simulink model "accelerometer02"  (R2016b)
settings: Solver=FixedStepAuto  StartTime=0.0  StopTime=inf  RelTol=1e-3
libraries: simulink_extras x2, androidlib x1
settings Model: SimulationMode=external  Creator=vibek  LastModifiedBy=vibek
settings OptimizationCC: MaxStackSize=64
settings DebuggingCC: ParameterTunabilityLossMsg=error
settings HardwareCC: ProdBitPerPointer=32  ProdBitPerSizeT=32  ProdBitPerPtrDiffT=32  ProdLargestAtomicInteger=Long  ProdLargestAtomicFloat=Double  ProdWordSize=32  ProdHWDeviceType=ARM Compatible->ARM Cortex  UseEmbeddedCoderFeatures=off  UseSimulinkCoderFeatures=off
settings RTWCC: SystemTargetFile=ert.tlc  HardwareBoard=Android Device  TLCOptions="-aInlineSetEventsForThisBaseRateFcn=TLC_FALSE -aSuppressMultiTaskScheduler=TLC_FALSE  -aRateBasedStepFcn=0"  TemplateMakefile=ert_default_tmf  Description=Embedded Coder  GenerateReport=on  Toolchain=Android SDK/NDK Tools  LaunchReport=on
settings CodeAppCC: ForceParamTrailComments=on  OperatorAnnotations=on  MATLABSourceComments=on
settings ERTTargetCC: ERTCustomFileBanners=off  SupportContinuousTime=on  SupportNonInlinedSFcns=on  RemoveResetFunc=off  ModelStepFunctionPrototypeControlCompliant=off

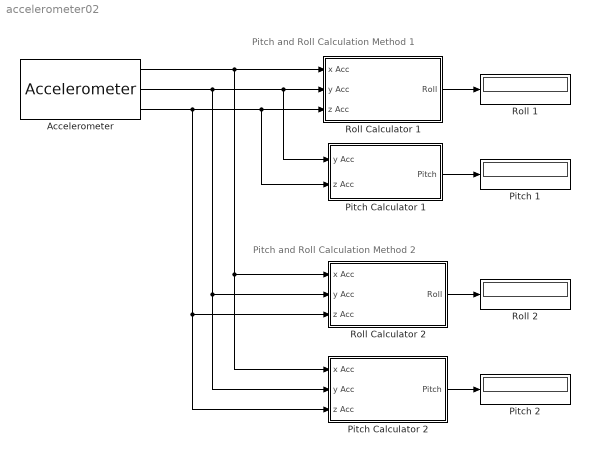
== system accelerometer02 ==
  note: Pitch and Roll Calculation Method 2
  note: Pitch and Roll Calculation Method 1
  Accelerometer : androidlib/Accelerometer  OutputVector=off  SampleTime=0.1  BlockPlatform=Android
  Pitch 1 : Display
      settings: Decimation=5
  Pitch 2 : Display
      settings: Decimation=6
  Pitch Calculator 1 : Subsystem
  Pitch Calculator 2 : Subsystem
  Roll 1 : Display
      settings: Decimation=5
  Roll 2 : Display
      settings: Decimation=6
  Roll Calculator 1 : Subsystem
  Roll Calculator 2 : Subsystem
  wires:
  Roll Calculator 1/1(Roll) -> Roll 1/1
  Pitch Calculator 1/1(Pitch) -> Pitch 1/1
  Accelerometer/1 -> Pitch Calculator 2/1(x Acc), Roll Calculator 2/1(x Acc), Roll Calculator 1/1(x Acc)
  Accelerometer/2 -> Pitch Calculator 2/2(y Acc), Roll Calculator 2/2(y Acc), Pitch Calculator 1/1(y Acc), Roll Calculator 1/2(y Acc)
  Accelerometer/3 -> Pitch Calculator 2/3(z Acc), Roll Calculator 2/3(z Acc), Pitch Calculator 1/2(z Acc), Roll Calculator 1/3(z Acc)
  Pitch Calculator 2/1(Pitch) -> Pitch 2/1
  Roll Calculator 2/1(Roll) -> Roll 2/1

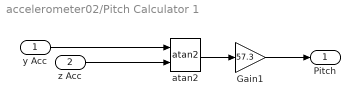
== system accelerometer02/Pitch Calculator 1 ==
  y Acc : Inport
  z Acc : Inport  Port=2
  Gain1 : Gain  Gain=57.3
  atan2 : Trigonometry  Operator=atan2
  Pitch : Outport
  wires:
  Gain1/1 -> Pitch/1
  atan2/1 -> Gain1/1
  y Acc/1 -> atan2/1
  z Acc/1 -> atan2/2

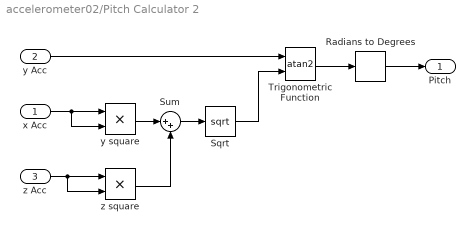
== system accelerometer02/Pitch Calculator 2 ==
  x Acc : Inport
  y Acc : Inport  Port=2
  z Acc : Inport  Port=3
  Radians to Degrees : simulink_extras/Transformations/Radians to Degrees
  Sqrt : Sqrt  SaturateOnIntegerOverflow=on
  Sum : Sum  Inputs=|++
  Trigonometric Function : Trigonometry  Operator=atan2
  y square : Product
  z square : Product
  Pitch : Outport
  wires:
  Radians to Degrees/1 -> Pitch/1
  Trigonometric Function/1 -> Radians to Degrees/1
  Sqrt/1 -> Trigonometric Function/2
  z square/1 -> Sum/2
  Sum/1 -> Sqrt/1
  z Acc/1 -> z square/1, z square/2
  y Acc/1 -> Trigonometric Function/1
  x Acc/1 -> y square/2, y square/1
  y square/1 -> Sum/1

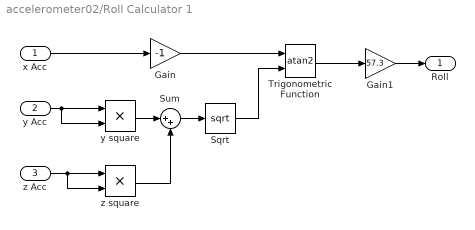
== system accelerometer02/Roll Calculator 1 ==
  x Acc : Inport
  y Acc : Inport  Port=2
  z Acc : Inport  Port=3
  Gain : Gain  Gain=-1
  Gain1 : Gain  Gain=57.3
  Sqrt : Sqrt  SaturateOnIntegerOverflow=on
  Sum : Sum  Inputs=|++
  Trigonometric Function : Trigonometry  Operator=atan2
  y square : Product
  z square : Product
  Roll : Outport
  wires:
  y Acc/1 -> y square/2, y square/1
  z Acc/1 -> z square/2, z square/1
  y square/1 -> Sum/1
  Sum/1 -> Sqrt/1
  z square/1 -> Sum/2
  x Acc/1 -> Gain/1
  Sqrt/1 -> Trigonometric Function/2
  Gain/1 -> Trigonometric Function/1
  Trigonometric Function/1 -> Gain1/1
  Gain1/1 -> Roll/1

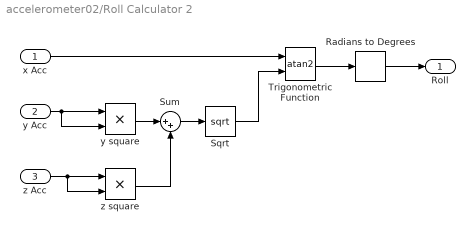
== system accelerometer02/Roll Calculator 2 ==
  x Acc : Inport
  y Acc : Inport  Port=2
  z Acc : Inport  Port=3
  Radians to Degrees : simulink_extras/Transformations/Radians to Degrees
  Sqrt : Sqrt  SaturateOnIntegerOverflow=on
  Sum : Sum  Inputs=|++
  Trigonometric Function : Trigonometry  Operator=atan2
  y square : Product
  z square : Product
  Roll : Outport
  wires:
  y Acc/1 -> y square/2, y square/1
  z Acc/1 -> z square/2, z square/1
  y square/1 -> Sum/1
  Sum/1 -> Sqrt/1
  z square/1 -> Sum/2
  Sqrt/1 -> Trigonometric Function/2
  x Acc/1 -> Trigonometric Function/1
  Trigonometric Function/1 -> Radians to Degrees/1
  Radians to Degrees/1 -> Roll/1
